simulink model "for_fft"  (R2016a)
settings: Solver=FixedStepAuto  StartTime=0.0  StopTime=time_array2(end)  FixedStep=Tstep  RelTol=1e-3
values from neighbouring files (symbols this model uses):
  Tstep = time_array(2) - time_array(1)    [series_unbalance_fft_analizleri.m]
libraries: powerlib x1
settings Model: Creator=mesutto  LastModifiedBy=mesutto

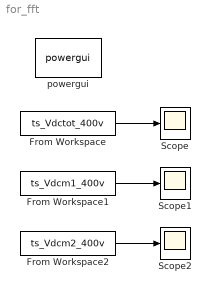
== system for_fft ==
  From Workspace : FromWorkspace  VariableName=ts_Vdctot_400v  SampleTime=Tstep
  From Workspace1 : FromWorkspace  VariableName=ts_Vdcm1_400v  SampleTime=Tstep
  From Workspace2 : FromWorkspace  VariableName=ts_Vdcm2_400v  SampleTime=Tstep
  Scope : Scope
  Scope1 : Scope
  Scope2 : Scope
  powergui : powerlib/powergui  Priority=1  SimulationMode=Discrete  SolverType=Tustin/Backward Euler (TBE)  SampleTime=Tstep  frequency=60  SPID=off  DisableSnubberDevices=off  DisableRonSwitches=off  DisableVfSwitches=off  SwTol=0  DisplayEquations=off  Interpol=off  ExternalGateDelay=off  methode=off  Ts=10  FunctionMessages=off  echomessages=off  HookPort=off  EnableUseOfTLC=off  x0status=blocks  frequencyindice=60  Pbase=100e6  ErrMax=1e-4  Iterations=50  UnitsV=kV  UnitsW=MW  buscounter=0  RestoreLinks=warning  ResistiveCurrentMeasurement=off  Frange=[0:2:500]  Ylog=off  Xlog=on  ShowGrid=off  save=off  variable=ZData  structure=0  ZoomFFT=off  StartTime=0.0  cycles=1  DisplayStyle=1  fundamental=60  FreqAxis=off  MaxFrequency=1000  frequencyindicesteady=1  RmsSteady=1  display=off
  wires:
  From Workspace/1 -> Scope/1
  From Workspace1/1 -> Scope1/1
  From Workspace2/1 -> Scope2/1
